simulink model "simulationclosedloop"  (R2021a)
settings: Solver=VariableStepAuto  StartTime=0.0  StopTime=100  RelTol=1e-3
values from neighbouring files (symbols this model uses):
  AA = [A0 zeros(3,1) ... (first row only)    [mainWithKxUncertainControl.m]
  Bua = [B; 0]    [mainWithKxUncertainControl.m]
  Bwa = [Bw; 0]    [mainWithKxUncertainControl.m]
  Ca = [C 0]    [mainWithKxUncertainControl.m]
  K = W*inv(P)    [mainWithKxUncertainControl.m]
settings Model: Creator=guilh  LastModifiedBy=guilh

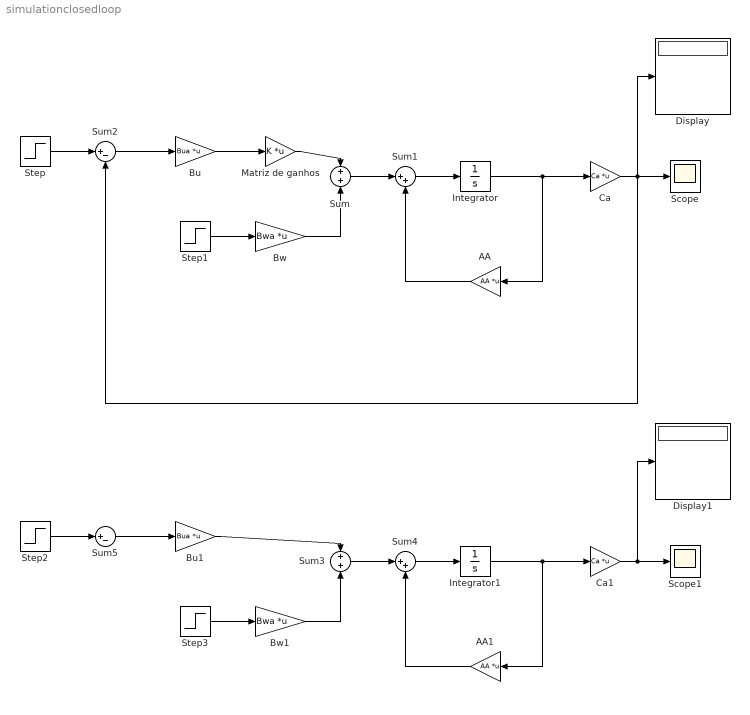
== system simulationclosedloop ==
  AA : Gain  Gain=AA  Multiplication=Matrix(K*u)
  AA1 : Gain  Gain=AA  Multiplication=Matrix(K*u)
  Bu : Gain  Gain=Bua  Multiplication=Matrix(K*u)
  Bu1 : Gain  Gain=Bua  Multiplication=Matrix(K*u)
  Bw : Gain  Gain=Bwa  Multiplication=Matrix(K*u)
  Bw1 : Gain  Gain=Bwa  Multiplication=Matrix(K*u)
  Ca : Gain  Gain=Ca  Multiplication=Matrix(K*u)
  Ca1 : Gain  Gain=Ca  Multiplication=Matrix(K*u)
  Display : Display
  Display1 : Display
  Integrator : Integrator
  Integrator1 : Integrator
  Matriz de ganhos : Gain  Gain=K  Multiplication=Matrix(K*u)
  Scope : Scope
  Scope1 : Scope
  Step : Step  SampleTime=0
  Step1 : Step  Time=5  After=0  SampleTime=0
  Step2 : Step  SampleTime=0
  Step3 : Step  Time=5  After=0  SampleTime=0
  Sum : Sum  Inputs=+|+
  Sum1 : Sum  Inputs=|++
  Sum2 : Sum  Inputs=|+-
  Sum3 : Sum  Inputs=+|+
  Sum4 : Sum  Inputs=|++
  Sum5 : Sum  Inputs=|+-
  wires:
  Bw/1 -> Sum/2
  AA/1 -> Sum1/2
  Ca/1 -> Display/1, Sum2/2, Scope/1
  Step/1 -> Sum2/1
  Step1/1 -> Bw/1
  Sum1/1 -> Integrator/1
  Integrator/1 -> AA/1, Ca/1
  Sum/1 -> Sum1/1
  Bu/1 -> Matriz de ganhos/1
  Matriz de ganhos/1 -> Sum/1
  Sum2/1 -> Bu/1
  Sum5/1 -> Bu1/1
  Integrator1/1 -> AA1/1, Ca1/1
  Sum4/1 -> Integrator1/1
  Sum3/1 -> Sum4/1
  Ca1/1 -> Display1/1, Scope1/1
  Step3/1 -> Bw1/1
  Bw1/1 -> Sum3/2
  Bu1/1 -> Sum3/1
  Step2/1 -> Sum5/1
  AA1/1 -> Sum4/2
